simulink model "DLQR_szimulink_model"  (R2018a)
settings: Solver=VariableStepAuto  StartTime=0.0  StopTime=10.0  RelTol=1e-3
values from neighbouring files (symbols this model uses):
  Adz = (Ad+Bd*K)    [DLQR_szabalyzo.m]
  Bdz = zeros(size(Bd))    [DLQR_szabalyzo.m]
  K = -inv(R+Bd'*P*Bd)*Bd'*P*Ad    [DLQR_szabalyzo.m]
  Ts = 0.2    [DLQR_szabalyzo.m]
  x0_mentett = x0    [DLQR_szabalyzo.m]
undefined symbols (not defined in the file or in its folder): Ad, Bd
settings Model: Creator=alfac  LastModifiedBy=alfac

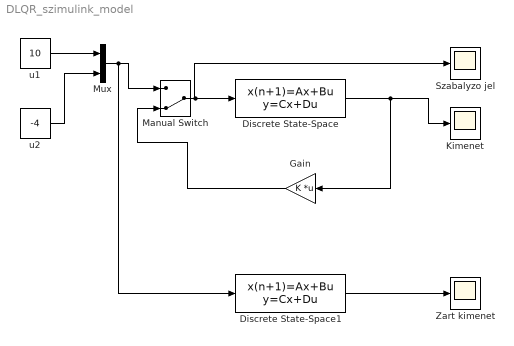
== system DLQR_szimulink_model ==
  Discrete State-Space : DiscreteStateSpace  A=Ad  B=Bd  C=eye(3)  D=zeros(3,2)  InitialCondition=x0_mentett  SampleTime=Ts
  Discrete State-Space1 : DiscreteStateSpace  A=Adz  B=Bdz  C=eye(3)  D=zeros(3,2)  InitialCondition=x0_mentett  SampleTime=Ts
  Gain : Gain  Gain=K  Multiplication=Matrix(K*u)
  "Kimenet " : Scope
  Manual Switch : ManualSwitch  CurrentSetting=0
  Mux : Mux  Inputs=2
  Szabalyzo jel : Scope
  Zart kimenet : Scope
  u1 : Constant  Value=10
  u2 : Constant  Value=-4
  wires:
  Discrete State-Space/1 -> "Kimenet "/1, Gain/1
  Gain/1 -> Manual Switch/2
  u1/1 -> Mux/1
  u2/1 -> Mux/2
  Mux/1 -> Discrete State-Space1/1, Manual Switch/1
  Manual Switch/1 -> Szabalyzo jel/1, Discrete State-Space/1
  Discrete State-Space1/1 -> Zart kimenet/1
